simulink model "problem1"  (R2020a)
settings: Solver=VariableStepAuto  StartTime=0.0  StopTime=10.0  RelTol=1e-3
settings Model: Creator=Riyansh  LastModifiedBy=Riyansh

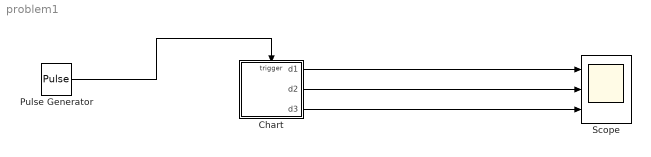
== system problem1 ==
  Chart : Stateflow chart  TreatAsAtomicUnit=on
  Pulse Generator : DiscretePulseGenerator  PulseType=Time based  Period=0.1  PulseWidth=5
  Scope : Scope  NumInputPorts=3
  wires:
  Chart/1(d1) -> Scope/1
  Chart/3(d3) -> Scope/3
  Chart/2(d2) -> Scope/2
  Pulse Generator/1 -> Chart/Trigger

== stateflow chart problem1/Chart ==
  settings: executeAtInitialization=1
  state digit1 [parallel]
    settings: executionOrder=1
    state One
      en:
      d1=1;
    state Two
      en:
      d1=2;
    state Zero
      en:
      d1=0;
    state Three
      en:
      d1=3;
    state Four
      en:
      d1=4;
    digit1.Two -> digit1.Three : inputClick
    digit1.Zero -> digit1.One : inputClick
    digit1.One -> digit1.Two : inputClick
    (default) -> digit1.Zero
    digit1.Four -> digit1.Zero : inputClick/{inc2}
    digit1.Three -> digit1.Four : inputClick
  state digit2 [parallel]
    settings: executionOrder=2
    state One
      en:
      d2=1;
    state Two
      en:
      d2=2;
    state Zero
      en:
      d2=0;
    state Three
      en:
      d2=3;
    state Four
      en:
      d2=4;
    digit2.Two -> digit2.Three : inc2
    digit2.Zero -> digit2.One : inc2
    digit2.One -> digit2.Two : inc2
    (default) -> digit2.Zero
    digit2.Four -> digit2.Zero : inc2/{inc3}
    digit2.Three -> digit2.Four : inc2
  state digit3 [parallel]
    settings: executionOrder=3
    state One
      en:
      d3=1;
    state Two
      en:
      d3=2;
    state Zero
      en:
      d3=0;
    state Three
      en:
      d3=3;
    state Four
      en:
      d3=4;
    digit3.Two -> digit3.Three : inc3
    digit3.Zero -> digit3.One : inc3
    digit3.One -> digit3.Two : inc3
    (default) -> digit3.Zero
    digit3.Four -> digit3.Zero : inc3
    digit3.Three -> digit3.Four : inc3
  (default) -> digit1
  data: d1 output; d2 output; d3 output
  events: inputClick input RISING_EDGE_EVENT; inc2 local RISING_EDGE_EVENT; inc3 local RISING_EDGE_EVENT
